simulink model "OpAmpDemo_original"  (R2021b)
settings: Solver=VariableStepAuto  StartTime=0.0  StopTime=inf  MaxStep=1e-4  RelTol=1e-3
libraries: ee_lib x22, fl_lib x18, nesl_utility x4
settings Model: PacingRate=0.010000  Creator=Work  LastModifiedBy=Work

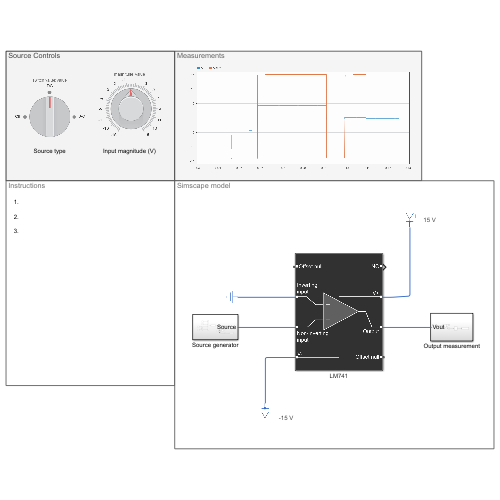
[thumbnail: Simulink's stored preview of the top-level diagram]
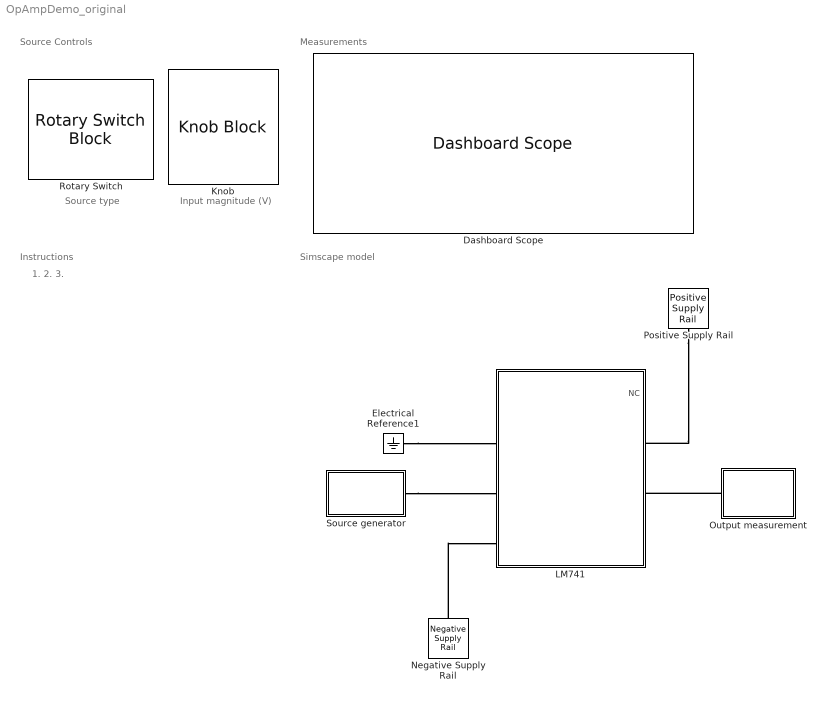
== system OpAmpDemo_original ==
  note: Input magnitude (V)
  note: Source type
  note: 1.
      |
      | 2.
      |
      | 3.
  note: Source Controls
  note: Measurements
  note: Simscape model
  note: Instructions
  Dashboard Scope : DashboardScope  TimeSpan=0.10000000000000001  Ymin=-16  Ymax=16  ScaleAtStop=off  UpdateMode=Scroll
  Electrical Reference1 : fl_lib/Electrical/Electrical Elements/Electrical Reference
  Knob : KnobBlock  ScaleMin=-15  ScaleMax=15
  LM741 : Subsystem
      mask Display: image('opampconnections.png');
  Negative Supply Rail : ee_lib/Sources/Negative Supply Rail  v0=-15 V
      settings: AttributesFormatString=%<v0> %<v0_unit>  SourceProductBaseCode=PS  InternalSimscapePortConfiguration="{\"Bottom\":[],\"Left\":[{\"id\":\"n\",\"label\":\"\",\"type\":\"foundation.electrical.electrical\"}],\"Right\":[],\"Top\":[]}"
  Output measurement : Subsystem
  Positive Supply Rail : ee_lib/Sources/Positive Supply Rail  v0=15 V
      settings: AttributesFormatString=%<v0> %<v0_unit>  SourceProductBaseCode=PS  InternalSimscapePortConfiguration="{\"Bottom\":[],\"Left\":[],\"Right\":[{\"id\":\"p\",\"label\":\"\",\"type\":\"foundation.electrical.electrical\"}],\"Top\":[]}"
  Rotary Switch : RotarySwitchBlock
      settings: Values={{'Off', 'DC', 'AC'}, [0 1 2]}
  Source generator : Subsystem
  connections:
  Electrical Reference1/LConn1 -- LM741/LConn2
  Source generator/RConn1 -- LM741/LConn3
  Output measurement/LConn1 -- LM741/RConn2
  Negative Supply Rail/LConn1 -- LM741/LConn4
  Positive Supply Rail/RConn1 -- LM741/RConn1

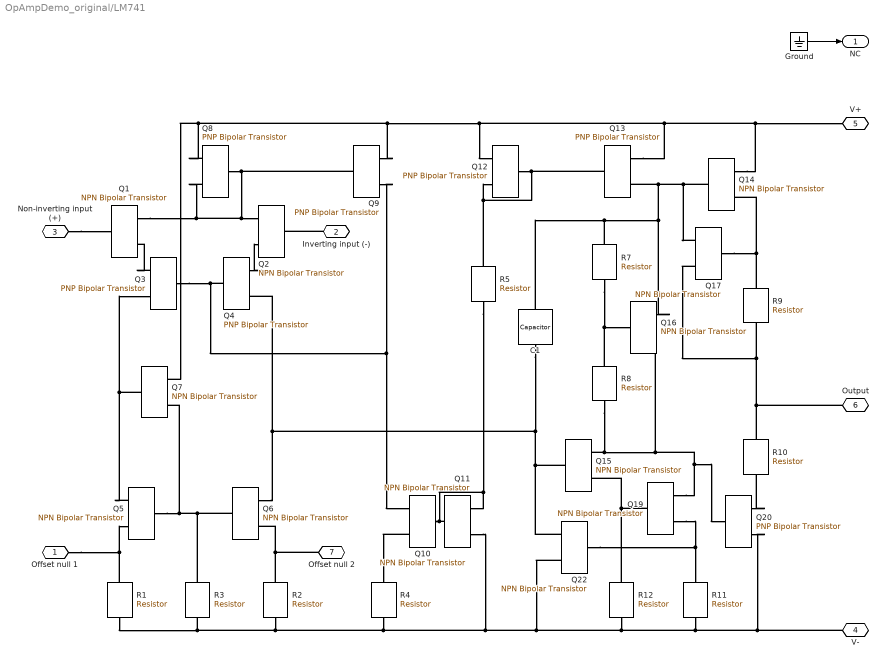
== system OpAmpDemo_original/LM741 ==
  C1 : fl_lib/Electrical/Electrical Elements/Capacitor  c=30 pF  r=1e-6 Ohm  g=0 1/Ohm  i_specify=off  i_priority=None  i=0 A  i_nominal_specify=off  i_nominal_unit=A  i_nominal_value=1  v_specify=off  v_priority=None  v=0 V  v_nominal_specify=off  v_nominal_unit=V  v_nominal_value=1  vc_specify=off  vc_priority=High  vc=0 V  vc_nominal_specify=off  vc_nominal_unit=V  vc_nominal_value=1
      settings: AttributesFormatString=%<c> %<c_unit>
  Ground : Ground
  Q{1..2,5..7,10..11,14..17,19,22} (13 alike) : ee_lib/Semiconductors & Converters/NPN Bipolar Transistor  parameterization=1  BF=100  IS=1e-14 A  VAF=200 V  hfe=100  hoe=50e-6 1/Ohm  Ic_h=1 mA  Vce_h=5 V  V1=0.55 V  I1=0.5 mA  BR=1  Tmeas=25 degC  RC=0.01 Ohm  RE=1e-4 Ohm  RB=1 Ohm  C_BC=5 pF  C_BE=5 pF  TF=0 us  TR=0 us  prmDatasheet=1  prmEquCoeff=1  hfe_T2=125  XTB=0  V1_T2=0.45 V  I1_T2=0.5 mA  Tmeas2=125 degC  EG=1.11 eV  XTI=3  TdeviceDatasheet=25 degC  TdeviceEquCoeff=25 degC  ec=1  thermal_network_parameterization=ee.enum.thermalNetworkTopology.junctionCase  Rth=[0, 10] K/W  Rth_Cauer=[1, 3, 10] K/W  Rth_Foster=[4, 6] K/W  thermal_mass_parameterization=ee.enum.thermalNetwork.timeconstant  thermal_mass=[0, 1] J/K  thermal_mass_Cauer=[.1, .3, 1] J/K  thermal_mass_Foster=[1.5, 3] J/K  thermal_time_constant=[0, 10] s  thermal_time_constant_Cauer=[1, 3, 10] s  thermal_time_constant_Foster=[6, 18] s  thermal_mass_initial_temperatures=[25, 25] degC  thermal_mass_initial_temperatures_Cauer=[25, 25, 25] degC  steadyState_Foster=simscape.enum.onoff.on  Tvec_initial_Foster=[25, 25, 25, 25] degC
  Q{3..4,8..9,12..13,20} (7 alike) : ee_lib/Semiconductors & Converters/PNP Bipolar Transistor  parameterization=1  BF=100  IS=1e-14 A  VAF=200 V  hfe=100  hoe=50e-6 1/Ohm  Ic_h=-1 mA  Vce_h=-5 V  V1=-0.55 V  I1=-0.5 mA  BR=1  Tmeas=25 degC  RC=0.01 Ohm  RE=1e-4 Ohm  RB=1 Ohm  C_BC=5 pF  C_BE=5 pF  TF=0 us  TR=0 us  prmDatasheet=1  prmEquCoeff=1  hfe_T2=125  XTB=0  V1_T2=-0.45 V  I1_T2=-0.5 mA  Tmeas2=125 degC  EG=1.11 eV  XTI=3  TdeviceDatasheet=25 degC  TdeviceEquCoeff=25 degC  ec=1  thermal_network_parameterization=ee.enum.thermalNetworkTopology.junctionCase  Rth=[0, 10] K/W  Rth_Cauer=[1, 3, 10] K/W  Rth_Foster=[4, 6] K/W  thermal_mass_parameterization=ee.enum.thermalNetwork.timeconstant  thermal_mass=[0, 1] J/K  thermal_mass_Cauer=[.1, .3, 1] J/K  thermal_mass_Foster=[1.5, 3] J/K  thermal_time_constant=[0, 10] s  thermal_time_constant_Cauer=[1, 3, 10] s  thermal_time_constant_Foster=[6, 18] s  thermal_mass_initial_temperatures=[25, 25] degC  thermal_mass_initial_temperatures_Cauer=[25, 25, 25] degC  steadyState_Foster=simscape.enum.onoff.on  Tvec_initial_Foster=[25, 25, 25, 25] degC
      settings: SourceProductBaseCode=PS  InternalSimscapePortConfiguration="{\"Bottom\":[],\"Left\":[{\"id\":\"B\",\"label\":\"\",\"type\":\"foundation.electrical.electrical\"}],\"Right\":[{\"id\":\"n\",\"label\":\"\",\"type\":\"foundation.electrical.electrical\"},{\"id\":\"p\",\"label\":\"\",\"type\":\"foundation.electrical.electrical\"}],\"Top\":[]}"
  R1 : fl_lib/Electrical/Electrical Elements/Resistor  R=1 kOhm  i_specify=off  i_priority=None  i=0 A  i_nominal_specify=off  i_nominal_unit=A  i_nominal_value=1  v_specify=off  v_priority=None  v=0 V  v_nominal_specify=off  v_nominal_unit=V  v_nominal_value=1
      settings: AttributesFormatString=%<R> %<R_unit>
  R10 : fl_lib/Electrical/Electrical Elements/Resistor  R=50 Ohm  i_specify=off  i_priority=None  i=0 A  i_nominal_specify=off  i_nominal_unit=A  i_nominal_value=1  v_specify=off  v_priority=None  v=0 V  v_nominal_specify=off  v_nominal_unit=V  v_nominal_value=1
      settings: AttributesFormatString=%<R> %<R_unit>
  R11 : fl_lib/Electrical/Electrical Elements/Resistor  R=50 Ohm  i_specify=off  i_priority=None  i=0 A  i_nominal_specify=off  i_nominal_unit=A  i_nominal_value=1  v_specify=off  v_priority=None  v=0 V  v_nominal_specify=off  v_nominal_unit=V  v_nominal_value=1
      settings: AttributesFormatString=%<R> %<R_unit>
  R12 : fl_lib/Electrical/Electrical Elements/Resistor  R=50 kOhm  i_specify=off  i_priority=None  i=0 A  i_nominal_specify=off  i_nominal_unit=A  i_nominal_value=1  v_specify=off  v_priority=None  v=0 V  v_nominal_specify=off  v_nominal_unit=V  v_nominal_value=1
      settings: AttributesFormatString=%<R> %<R_unit>
  R2 : fl_lib/Electrical/Electrical Elements/Resistor  R=1 kOhm  i_specify=off  i_priority=None  i=0 A  i_nominal_specify=off  i_nominal_unit=A  i_nominal_value=1  v_specify=off  v_priority=None  v=0 V  v_nominal_specify=off  v_nominal_unit=V  v_nominal_value=1
      settings: AttributesFormatString=%<R> %<R_unit>
  R3 : fl_lib/Electrical/Electrical Elements/Resistor  R=50 kOhm  i_specify=off  i_priority=None  i=0 A  i_nominal_specify=off  i_nominal_unit=A  i_nominal_value=1  v_specify=off  v_priority=None  v=0 V  v_nominal_specify=off  v_nominal_unit=V  v_nominal_value=1
      settings: AttributesFormatString=%<R> %<R_unit>
  R4 : fl_lib/Electrical/Electrical Elements/Resistor  R=5 kOhm  i_specify=off  i_priority=None  i=0 A  i_nominal_specify=off  i_nominal_unit=A  i_nominal_value=1  v_specify=off  v_priority=None  v=0 V  v_nominal_specify=off  v_nominal_unit=V  v_nominal_value=1
      settings: AttributesFormatString=%<R> %<R_unit>
  R5 : fl_lib/Electrical/Electrical Elements/Resistor  R=39 kOhm  i_specify=off  i_priority=None  i=0 A  i_nominal_specify=off  i_nominal_unit=A  i_nominal_value=1  v_specify=off  v_priority=None  v=0 V  v_nominal_specify=off  v_nominal_unit=V  v_nominal_value=1
      settings: AttributesFormatString=%<R> %<R_unit>
  R7 : fl_lib/Electrical/Electrical Elements/Resistor  R=4.5 kOhm  i_specify=off  i_priority=None  i=0 A  i_nominal_specify=off  i_nominal_unit=A  i_nominal_value=1  v_specify=off  v_priority=None  v=0 V  v_nominal_specify=off  v_nominal_unit=V  v_nominal_value=1
      settings: AttributesFormatString=%<R> %<R_unit>
  R8 : fl_lib/Electrical/Electrical Elements/Resistor  R=7.5 kOhm  i_specify=off  i_priority=None  i=0 A  i_nominal_specify=off  i_nominal_unit=A  i_nominal_value=1  v_specify=off  v_priority=None  v=0 V  v_nominal_specify=off  v_nominal_unit=V  v_nominal_value=1
      settings: AttributesFormatString=%<R> %<R_unit>
  R9 : fl_lib/Electrical/Electrical Elements/Resistor  R=25 Ohm  i_specify=off  i_priority=None  i=0 A  i_nominal_specify=off  i_nominal_unit=A  i_nominal_value=1  v_specify=off  v_priority=None  v=0 V  v_nominal_specify=off  v_nominal_unit=V  v_nominal_value=1
      settings: AttributesFormatString=%<R> %<R_unit>
  Offset null 1 : PMIOPort  Side=Left
  Inverting input (-) : PMIOPort  Port=2  Side=Left
  Non-inverting input (+) : PMIOPort  Port=3  Side=Left
  V- : PMIOPort  Port=4  Side=Left
  V+ : PMIOPort  Port=5  Side=Right
  Output : PMIOPort  Port=6  Side=Right
  Offset null 2 : PMIOPort  Port=7  Side=Right
  NC : Outport
  wires:
  Ground/1 -> NC/1
  connections:
  Q6/RConn1 -- Q15/LConn1 -- Q22/RConn1 -- C1/RConn1 -- Q4/RConn2
  R1/RConn1 -- V-/RConn1 -- Q20/RConn2 -- R11/RConn1 -- R12/RConn1 -- Q22/RConn2 -- Q11/RConn2 -- R4/RConn1 -- R2/RConn1 -- R3/RConn1
  Q1/RConn1 -- Q9/LConn1 -- Q8/LConn1 -- Q2/RConn1 -- Q8/RConn2
  Q14/LConn1 -- Q17/RConn1 -- C1/LConn1 -- R7/LConn1 -- Q16/RConn1 -- Q13/RConn2
  R2/LConn1 -- Offset null 2/RConn1 -- Q6/RConn2
  Q3/LConn1 -- Q4/LConn1 -- Q9/RConn2 -- Q10/RConn1
  Q9/RConn1 -- Q12/RConn1 -- Q13/RConn1 -- V+/RConn1 -- Q14/RConn1 -- Q8/RConn1 -- Q7/RConn1
  Q7/LConn1 -- Q5/RConn1 -- Q3/RConn2
  Q4/RConn1 -- Q2/RConn2
  Q19/RConn1 -- R8/RConn1 -- Q15/RConn1 -- Q16/RConn2 -- Q20/LConn1
  Q20/RConn1 -- R10/RConn1
  Q17/LConn1 -- R9/LConn1 -- Q14/RConn2
  Q10/RConn2 -- R4/LConn1
  Q17/RConn2 -- Output/RConn1 -- R10/LConn1 -- R9/RConn1
  R5/LConn1 -- Q13/LConn1 -- Q12/LConn1 -- Q12/RConn2
  Q19/LConn1 -- R12/LConn1 -- Q15/RConn2
  Q11/LConn1 -- Q10/LConn1 -- R5/RConn1 -- Q11/RConn1
  Q19/RConn2 -- Q22/LConn1 -- R11/LConn1
  Non-inverting input (+)/RConn1 -- Q1/LConn1
  R7/RConn1 -- R8/LConn1 -- Q16/LConn1
  Q5/LConn1 -- R3/LConn1 -- Q6/LConn1 -- Q7/RConn2
  R1/LConn1 -- Offset null 1/RConn1 -- Q5/RConn2
  Inverting input (-)/RConn1 -- Q2/LConn1
  Q3/RConn1 -- Q1/RConn2

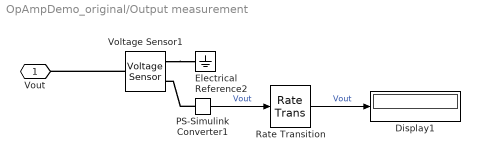
== system OpAmpDemo_original/Output measurement ==
  Display1 : Display
  Electrical Reference2 : fl_lib/Electrical/Electrical Elements/Electrical Reference
  PS-Simulink Converter1 : nesl_utility/PS-Simulink Converter  PhysicalDomain=network_engine_domain  SubClassName=ps_output  LeftPortType=input  RightPortType=output  PseudoPeriodic=off  Frequencies=[]  Unit=inherit  AffineConversion=off
      settings: SourceProductBaseCode=PW,SS
  Rate Transition : RateTransition  OutPortSampleTime=0.0001
  Voltage Sensor1 : fl_lib/Electrical/Electrical Sensors/Voltage Sensor
  Vout : PMIOPort  Side=Left
  wires:
  PS-Simulink Converter1/1 -> Rate Transition/1  "Vout"
  Rate Transition/1 -> Display1/1  "Vout"
  connections:
  Voltage Sensor1/LConn1 -- Vout/RConn1
  Voltage Sensor1/RConn2 -- Electrical Reference2/LConn1
  PS-Simulink Converter1/LConn1 -- Voltage Sensor1/RConn1

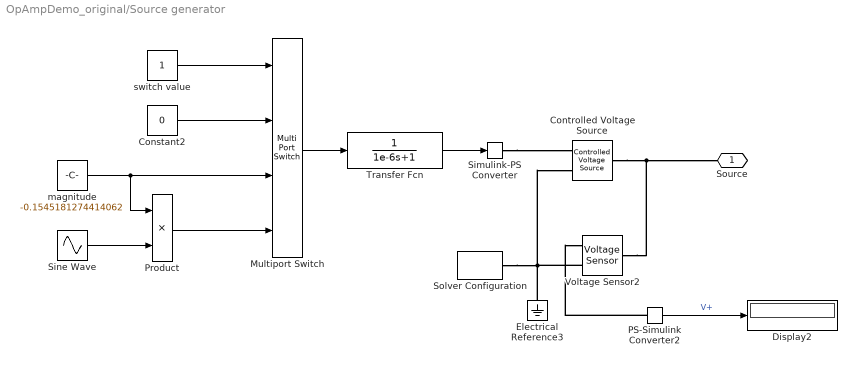
== system OpAmpDemo_original/Source generator ==
  Constant2 : Constant  Value=0
  Controlled Voltage Source : fl_lib/Electrical/Electrical Sources/Controlled Voltage Source
  Display2 : Display
  Electrical Reference3 : fl_lib/Electrical/Electrical Elements/Electrical Reference
  Multiport Switch : MultiPortSwitch  DataPortOrder=Zero-based contiguous  zeroidx=on
  PS-Simulink Converter2 : nesl_utility/PS-Simulink Converter  PhysicalDomain=network_engine_domain  SubClassName=ps_output  LeftPortType=input  RightPortType=output  PseudoPeriodic=off  Frequencies=[]  Unit=inherit  AffineConversion=off
      settings: SourceProductBaseCode=PW,SS
  Product : Product
  Simulink-PS Converter : nesl_utility/Simulink-PS Converter  PhysicalDomain=network_engine_domain  SubClassName=ps_input  LeftPortType=input  RightPortType=output  PseudoPeriodic=off  Frequencies=[]  NoiseDistribution=none  NoiseParameters=[]  Unit=1  AffineConversion=off  FilteringAndDerivatives=provide  SimscapeFilterOrder=1  InputFilterTimeConstant=0.001  UdotUserProvided=0
      settings: SourceProductBaseCode=PW,SS
  Sine Wave : Sin  Frequency=2*pi*60  SampleTime=0
  Solver Configuration : nesl_utility/Solver Configuration  PhysicalDomain=network_engine_domain  SubClassName=solver  LeftPortType=input  RightPortType=generic  Tones=[]  Harmonics=[]  SimulateNoise=off  Profile=off  UseLocalSampling=off  EnableSwitchedLinearOptims=on  FrequencyDomain=off  UseCCode=off  RelTol=0.001  AbsTol=1e-06  MinStep=1e-09  ToWorkspace=off  RevertToSquareIcSolve=off  NumHomotopyIterations=100  PhasorMode=off  PhasorModeNumHarmonics=1  DoDC=off  ResidualTolerance=1e-09  UseLocalSolver=off  LocalSolverChoice=NE_BACKWARD_EULER_ADVANCER  LocalSolverSampleTime=0.001  DoFixedCost=off  MaxNonlinIter=3  MaxModeIter=2  ComputeImpulses=off  ImpulseIterations=2  LinearAlgebra=auto  EquationFormulation=NE_TIME_EF  DelaysMemoryBudget=1024  AutomaticFiltering=on  FilteringTimeConstant=0.001  PartitionStorageMethod=AS_NEEDED  PartitionMemoryBudget=1024  PartitionMethod=ROBUST
      settings: SourceProductBaseCode=PW,SS
  Transfer Fcn : TransferFcn  Denominator=[1e-6 1]
  Voltage Sensor2 : fl_lib/Electrical/Electrical Sensors/Voltage Sensor
  magnitude : Constant  Value=-0.1545181274414062
  switch value : Constant
  Source : PMIOPort  Side=Right
  wires:
  PS-Simulink Converter2/1 -> Display2/1  "V+"
  Sine Wave/1 -> Product/2
  magnitude/1 -> Multiport Switch/3, Product/1
  Product/1 -> Multiport Switch/4
  Multiport Switch/1 -> Transfer Fcn/1
  switch value/1 -> Multiport Switch/1
  Constant2/1 -> Multiport Switch/2
  Transfer Fcn/1 -> Simulink-PS Converter/1
  connections:
  Electrical Reference3/LConn1 -- Solver Configuration/RConn1 -- Controlled Voltage Source/RConn2 -- Voltage Sensor2/RConn2
  Controlled Voltage Source/LConn1 -- Voltage Sensor2/LConn1 -- Source/RConn1
  PS-Simulink Converter2/LConn1 -- Voltage Sensor2/RConn1
  Simulink-PS Converter/RConn1 -- Controlled Voltage Source/RConn1
